simulink model "QPSK_sim"  (R2016b)
settings: Solver=ode45  StartTime=0  StopTime=L  MaxStep=1  RelTol=1e-3  EnableMultiTasking=on
values from neighbouring files (symbols this model uses):
  Beta = 0.2    [QPSK.m]
  BW_LPF = BW_CH*60    (= 0.46875)    [QPSK.m]
  C_aprox = [1.60695392426680e-05 2.95841123026030e-05 5.48262790927617e-05 9.19832588239474e-05 0.000143686658983094 0.000212359882657570 0.000299965229015387 0.000407761225657029 0.000536071876123679 0.000684099631525166 0.000849796105711060 0.00102983168952252 0.00121960996869630 0.00141347333081234 0.00160490224533182 0.00178687182515771 0.00195224251942712 0.00209417001193910 0.00220655685058343 0.002284 ...(+463 chars)    [QPSK.m]
  fc = fe/4    (= 0.25)    [QPSK.m]
  Samples_N = Tsymb/Te    [QPSK.m]
  sin_amp = 1    [QPSK.m]
  Te = 1/fe    (= 1)    [QPSK.m]
  Tsymb = round((1/BW_CH)*(1+Beta)*Te/2)    [QPSK.m]
undefined symbols (not defined in the file or in its folder): a, b, c, g
libraries: commfilt2 x2, commrandsrc2 x2
settings Model: Creator=Solomesta  LastModifiedBy=charles
settings DataIOCC: LimitDataPoints=on  SaveFormat=Array
settings OptimizationCC: LifeSpan=inf
settings DebuggingCC: SolverPrmCheckMsg=warning  SFUnexpectedBacktrackingDiag=warning  SFNoUnconditionalDefaultTransitionDiag=warning  SFExecutionAtInitializationDiag=none
settings HardwareCC: ProdBitPerPointer=32  ProdBitPerSizeT=32  ProdBitPerPtrDiffT=32  ProdLargestAtomicFloat=None  ProdIntDivRoundTo=Undefined  ProdEndianess=Unspecified  ProdWordSize=32  ProdHWDeviceType=32-bit Generic
settings ModelReferenceCC: PropagateSignalLabelsOutOfModel=off
settings GRTTargetCC: TargetLangStandard=C89/C90 (ANSI)  GeneratePreprocessorConditionals=Disable all
settings ConfigComp: CovMetricSettings=dw  CovHtmlReporting=on  CovSaveCumulativeToWorkspaceVar=on  CovSaveSingleToWorkspaceVar=on  CovExternalEMLEnable=off  CovSFcnEnable=off

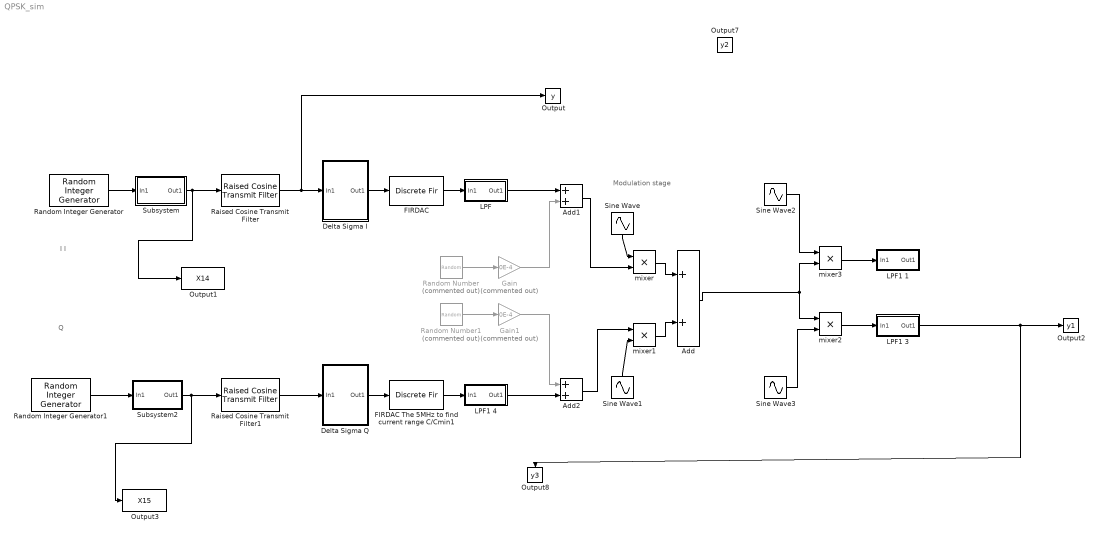
== system QPSK_sim ==
  note: Modulation stage
  note: Q
  note: I
      | I
  " LPF " : Subsystem
  " LPF1 1" : Subsystem
  " LPF1 3" : Subsystem
  " LPF1 4" : Subsystem
  Add : Sum
  Add1 : Sum
  Add2 : Sum
  Delta Sigma I : Subsystem
  "Delta Sigma Q " : Subsystem
  "FIRDAC " : DiscreteFir  Tag=BlockMethodSubSystem  Coefficients=C_aprox  InputProcessing=Columns as channels (frame based)  SampleTime=Te
  FIRDAC The 5MHz to find current range C/Cmin1 : DiscreteFir  Tag=BlockMethodSubSystem  Coefficients=C_aprox  InputProcessing=Columns as channels (frame based)  SampleTime=Te
  Gain : Gain  Commented=on  Gain=0E-4
  Gain1 : Gain  Commented=on  Gain=0E-4
  Output : ToWorkspace  VariableName=y  SaveFormat=Structure With Time  SampleTime=1
      settings: MaxDataPoints=N
  Output1 : ToWorkspace  VariableName=X14  SaveFormat=Structure With Time  SampleTime=Te
      settings: MaxDataPoints=N
  Output2 : ToWorkspace  VariableName=y1  SaveFormat=Structure With Time  SampleTime=1
      settings: MaxDataPoints=N
  Output3 : ToWorkspace  VariableName=X15  SaveFormat=Structure With Time  SampleTime=Te
      settings: MaxDataPoints=N
  Output7 : ToWorkspace  VariableName=y2  SaveFormat=Structure With Time  SampleTime=Te
      settings: MaxDataPoints=N
  Output8 : ToWorkspace  VariableName=y3  SaveFormat=Structure With Time  SampleTime=Te
      settings: MaxDataPoints=N
  Raised Cosine Transmit Filter : commfilt2/Raised Cosine Transmit Filter  filtType=Normal  R=Beta  filtSpan=2  N=Samples_N  filterGain=1  InputProcessing=Columns as channels (frame based)  RateOptions=Allow multirate processing  framing=Mute  checkCoeff=off  variableName=rcTxFilt  checkGain=Normalized  sampMode=Mute  saveAsFlag=0  currentFiltSpan=2  D=(2)/2  launchFVT=on  roundingMode=Floor  overflowMode=off  coeffDataTypeStr=Inherit: Same word length as input  coeffMin=[]  coeffMax=[]  coeffLastDataTypeStr=Inherit: Same word length as input  outputDataTypeStr=Inherit: Same as accumulator  outputMin=[]  outputMax=[]  outputLastDataTypeStr=Inherit: Same as accumulator
  Raised Cosine Transmit Filter1 : commfilt2/Raised Cosine Transmit Filter  filtType=Normal  R=Beta  filtSpan=2  N=Samples_N  filterGain=1  InputProcessing=Columns as channels (frame based)  RateOptions=Allow multirate processing  framing=Mute  checkCoeff=off  variableName=rcTxFilt1  checkGain=Normalized  sampMode=Mute  saveAsFlag=0  currentFiltSpan=2  D=(2)/2  launchFVT=on  roundingMode=Floor  overflowMode=off  coeffDataTypeStr=Inherit: Same word length as input  coeffMin=[]  coeffMax=[]  coeffLastDataTypeStr=Inherit: Same word length as input  outputDataTypeStr=Inherit: Same as accumulator  outputMin=[]  outputMax=[]  outputLastDataTypeStr=Inherit: Same as accumulator
  Random Number : RandomNumber  Commented=on  Seed=26  SampleTime=Te
  Random Number1 : RandomNumber  Commented=on  Seed=26  SampleTime=Te
  Random Integer Generator : commrandsrc2/Random Integer Generator  mul=2  seed=37  Ts=Tsymb  frameBased=off  sampPerFrame=1  orient=off  outDataType=double
  Random Integer Generator1 : commrandsrc2/Random Integer Generator  mul=2  seed=3000  Ts=Tsymb  frameBased=off  sampPerFrame=1  orient=off  outDataType=double
  Sine Wave : Sin  Amplitude=sin_amp  Frequency=fc*2*pi  Samples=4  SampleTime=Te
  Sine Wave1 : Sin  Amplitude=sin_amp  Frequency=fc*2*pi  Phase=pi/2  SampleTime=Te
  Sine Wave2 : Sin  Amplitude=sin_amp  Frequency=fc*2*pi  SampleTime=Te
  Sine Wave3 : Sin  Amplitude=sin_amp  Frequency=fc*2*pi  Phase=pi/2  SampleTime=Te
  Subsystem : Subsystem
  Subsystem2 : Subsystem
  mixer{,1..3} (4 alike) : Product  Inputs=**
  wires:
  Random Integer Generator/1 -> Subsystem/1(In1)
  Delta Sigma I/1(Out1) -> "FIRDAC "/1
  Sine Wave/1 -> mixer/1
  Random Integer Generator1/1 -> Subsystem2/1(In1)
  "Delta Sigma Q "/1(Out1) -> FIRDAC The 5MHz to find current range C/Cmin1/1
  mixer1/1 -> Add/2
  "FIRDAC "/1 -> " LPF "/1(In1)
  Add/1 -> mixer3/2, mixer2/1
  Sine Wave3/1 -> mixer2/2
  Sine Wave2/1 -> mixer3/1
  mixer/1 -> Add/1
  FIRDAC The 5MHz to find current range C/Cmin1/1 -> " LPF1 4"/1(In1)
  Add1/1 -> mixer/2
  Random Number/1 -> Gain/1
  Sine Wave1/1 -> mixer1/2
  Raised Cosine Transmit Filter/1 -> Output/1, Delta Sigma I/1(In1)
  Raised Cosine Transmit Filter1/1 -> "Delta Sigma Q "/1(In1)
  mixer3/1 -> " LPF1 1"/1(In1)
  mixer2/1 -> " LPF1 3"/1(In1)
  " LPF "/1(Out1) -> Add1/1
  " LPF1 4"/1(Out1) -> Add2/2
  Add2/1 -> mixer1/1
  Random Number1/1 -> Gain1/1
  Gain/1 -> Add1/2
  Gain1/1 -> Add2/1
  Subsystem/1(Out1) -> Output1/1, Raised Cosine Transmit Filter/1
  Subsystem2/1(Out1) -> Output3/1, Raised Cosine Transmit Filter1/1
  " LPF1 3"/1(Out1) -> Output8/1, Output2/1

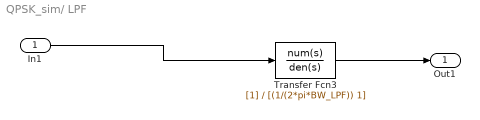
== system QPSK_sim/ LPF  ==
  In1 : Inport
  Transfer Fcn3 : TransferFcn  Denominator=[(1/(2*pi*BW_LPF)) 1]
  Out1 : Outport
  wires:
  In1/1 -> Transfer Fcn3/1
  Transfer Fcn3/1 -> Out1/1

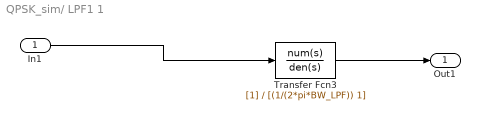
== system QPSK_sim/ LPF1 1 ==
  In1 : Inport
  Transfer Fcn3 : TransferFcn  Denominator=[(1/(2*pi*BW_LPF)) 1]
  Out1 : Outport
  wires:
  In1/1 -> Transfer Fcn3/1
  Transfer Fcn3/1 -> Out1/1

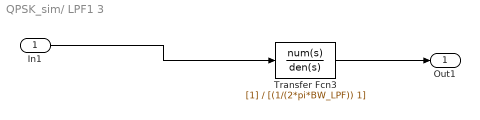
== system QPSK_sim/ LPF1 3 ==
  In1 : Inport
  Transfer Fcn3 : TransferFcn  Denominator=[(1/(2*pi*BW_LPF)) 1]
  Out1 : Outport
  wires:
  In1/1 -> Transfer Fcn3/1
  Transfer Fcn3/1 -> Out1/1

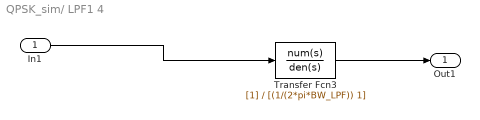
== system QPSK_sim/ LPF1 4 ==
  In1 : Inport
  Transfer Fcn3 : TransferFcn  Denominator=[(1/(2*pi*BW_LPF)) 1]
  Out1 : Outport
  wires:
  In1/1 -> Transfer Fcn3/1
  Transfer Fcn3/1 -> Out1/1

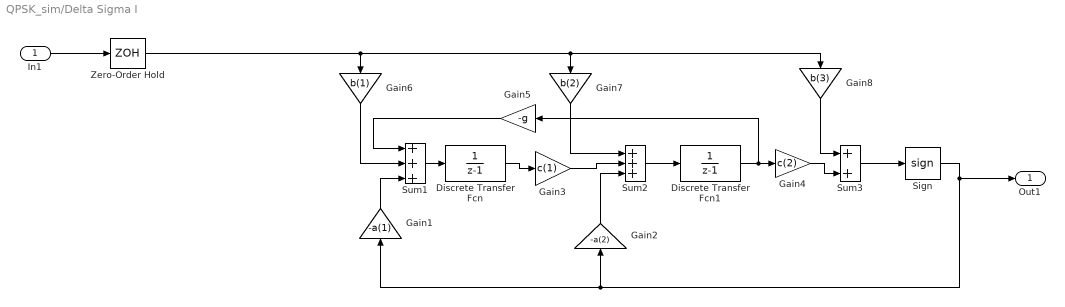
== system QPSK_sim/Delta Sigma I ==
  In1 : Inport
  Discrete Transfer Fcn : DiscreteTransferFcn  Denominator=[1 -1]
  Discrete Transfer Fcn1 : DiscreteTransferFcn  Denominator=[1 -1]
  Gain1 : Gain  Gain=-a(1)  SaturateOnIntegerOverflow=on  OutDataTypeStr=Inherit: Same as input  ParamDataTypeStr=Inherit: Same as input
  Gain2 : Gain  Gain=-a(2)  SaturateOnIntegerOverflow=on  OutDataTypeStr=Inherit: Same as input  ParamDataTypeStr=Inherit: Same as input
  Gain3 : Gain  Gain=c(1)  SaturateOnIntegerOverflow=on  OutDataTypeStr=Inherit: Same as input  ParamDataTypeStr=Inherit: Same as input
  Gain4 : Gain  Gain=c(2)  SaturateOnIntegerOverflow=on  OutDataTypeStr=Inherit: Same as input  ParamDataTypeStr=Inherit: Same as input
  Gain5 : Gain  Gain=-g  SaturateOnIntegerOverflow=on  OutDataTypeStr=Inherit: Same as input  ParamDataTypeStr=Inherit: Same as input
  Gain6 : Gain  Gain=b(1)  SaturateOnIntegerOverflow=on  OutDataTypeStr=Inherit: Same as input  ParamDataTypeStr=Inherit: Same as input
  Gain7 : Gain  Gain=b(2)  SaturateOnIntegerOverflow=on  OutDataTypeStr=Inherit: Same as input  ParamDataTypeStr=Inherit: Same as input
  Gain8 : Gain  Gain=b(3)  SaturateOnIntegerOverflow=on  OutDataTypeStr=Inherit: Same as input  ParamDataTypeStr=Inherit: Same as input
  Sign : Signum
  Sum1 : Sum  Inputs=+++  SaturateOnIntegerOverflow=on  InputSameDT=on  OutDataTypeStr=Inherit: Same as first input
  Sum2 : Sum  Inputs=+++  SaturateOnIntegerOverflow=on  InputSameDT=on  OutDataTypeStr=Inherit: Same as first input
  Sum3 : Sum  SaturateOnIntegerOverflow=on  InputSameDT=on  OutDataTypeStr=Inherit: Same as first input
  Zero-Order Hold : ZeroOrderHold  SampleTime=Te
  Out1 : Outport
  wires:
  In1/1 -> Zero-Order Hold/1
  Discrete Transfer Fcn1/1 -> Gain5/1, Gain4/1
  Gain8/1 -> Sum3/1
  Gain2/1 -> Sum2/3
  Sum3/1 -> Sign/1
  Gain1/1 -> Sum1/3
  Gain7/1 -> Sum2/1
  Sum2/1 -> Discrete Transfer Fcn1/1
  Gain4/1 -> Sum3/2
  Gain3/1 -> Sum2/2
  Sign/1 -> Out1/1, Gain1/1, Gain2/1
  Discrete Transfer Fcn/1 -> Gain3/1
  Gain5/1 -> Sum1/1
  Gain6/1 -> Sum1/2
  Sum1/1 -> Discrete Transfer Fcn/1
  Zero-Order Hold/1 -> Gain6/1, Gain8/1, Gain7/1

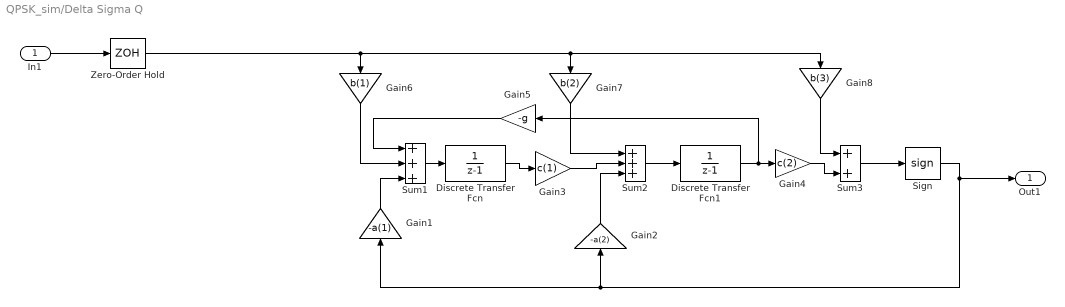
== system QPSK_sim/Delta Sigma Q  ==
  In1 : Inport
  Discrete Transfer Fcn : DiscreteTransferFcn  Denominator=[1 -1]
  Discrete Transfer Fcn1 : DiscreteTransferFcn  Denominator=[1 -1]
  Gain1 : Gain  Gain=-a(1)  SaturateOnIntegerOverflow=on  OutDataTypeStr=Inherit: Same as input  ParamDataTypeStr=Inherit: Same as input
  Gain2 : Gain  Gain=-a(2)  SaturateOnIntegerOverflow=on  OutDataTypeStr=Inherit: Same as input  ParamDataTypeStr=Inherit: Same as input
  Gain3 : Gain  Gain=c(1)  SaturateOnIntegerOverflow=on  OutDataTypeStr=Inherit: Same as input  ParamDataTypeStr=Inherit: Same as input
  Gain4 : Gain  Gain=c(2)  SaturateOnIntegerOverflow=on  OutDataTypeStr=Inherit: Same as input  ParamDataTypeStr=Inherit: Same as input
  Gain5 : Gain  Gain=-g  SaturateOnIntegerOverflow=on  OutDataTypeStr=Inherit: Same as input  ParamDataTypeStr=Inherit: Same as input
  Gain6 : Gain  Gain=b(1)  SaturateOnIntegerOverflow=on  OutDataTypeStr=Inherit: Same as input  ParamDataTypeStr=Inherit: Same as input
  Gain7 : Gain  Gain=b(2)  SaturateOnIntegerOverflow=on  OutDataTypeStr=Inherit: Same as input  ParamDataTypeStr=Inherit: Same as input
  Gain8 : Gain  Gain=b(3)  SaturateOnIntegerOverflow=on  OutDataTypeStr=Inherit: Same as input  ParamDataTypeStr=Inherit: Same as input
  Sign : Signum
  Sum1 : Sum  Inputs=+++  SaturateOnIntegerOverflow=on  InputSameDT=on  OutDataTypeStr=Inherit: Same as first input
  Sum2 : Sum  Inputs=+++  SaturateOnIntegerOverflow=on  InputSameDT=on  OutDataTypeStr=Inherit: Same as first input
  Sum3 : Sum  SaturateOnIntegerOverflow=on  InputSameDT=on  OutDataTypeStr=Inherit: Same as first input
  Zero-Order Hold : ZeroOrderHold  SampleTime=Te
  Out1 : Outport
  wires:
  In1/1 -> Zero-Order Hold/1
  Discrete Transfer Fcn1/1 -> Gain5/1, Gain4/1
  Gain8/1 -> Sum3/1
  Gain2/1 -> Sum2/3
  Sum3/1 -> Sign/1
  Gain1/1 -> Sum1/3
  Gain7/1 -> Sum2/1
  Sum2/1 -> Discrete Transfer Fcn1/1
  Gain4/1 -> Sum3/2
  Gain3/1 -> Sum2/2
  Sign/1 -> Out1/1, Gain1/1, Gain2/1
  Discrete Transfer Fcn/1 -> Gain3/1
  Gain5/1 -> Sum1/1
  Gain6/1 -> Sum1/2
  Sum1/1 -> Discrete Transfer Fcn/1
  Zero-Order Hold/1 -> Gain6/1, Gain8/1, Gain7/1

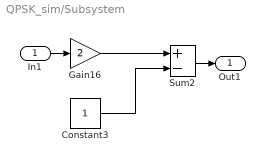
== system QPSK_sim/Subsystem ==
  In1 : Inport
  Constant3 : Constant  SampleTime=-1
  Gain16 : Gain  Gain=2
  Sum2 : Sum  Inputs=+-  SaturateOnIntegerOverflow=on  InputSameDT=on  OutDataTypeStr=Inherit: Same as first input
  Out1 : Outport
  wires:
  Constant3/1 -> Sum2/2
  Gain16/1 -> Sum2/1
  Sum2/1 -> Out1/1
  In1/1 -> Gain16/1

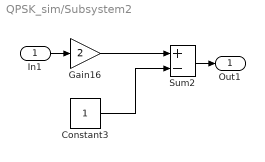
== system QPSK_sim/Subsystem2 ==
  In1 : Inport
  Constant3 : Constant  SampleTime=-1
  Gain16 : Gain  Gain=2
  Sum2 : Sum  Inputs=+-  SaturateOnIntegerOverflow=on  InputSameDT=on  OutDataTypeStr=Inherit: Same as first input
  Out1 : Outport
  wires:
  Constant3/1 -> Sum2/2
  Gain16/1 -> Sum2/1
  Sum2/1 -> Out1/1
  In1/1 -> Gain16/1
